simulink subsystem "sensorModels"  (R2026a)
settings: Solver=VariableStepAuto
values from neighbouring files (symbols this model uses):
  envParams : value not decoded    [plantParams.sldd]
  sensorParams : value not decoded    [plantParams.sldd]
undefined symbols (not defined in the file or in its folder): WMM2025
libraries: simulink x7, matrix_library x3, aerolibgravity2 x1
settings Model: DataDictionary=plantParams.sldd  EnableAccessToBaseWorkspace=off  Creator=nathanscott  LastModifiedBy=nathanscott

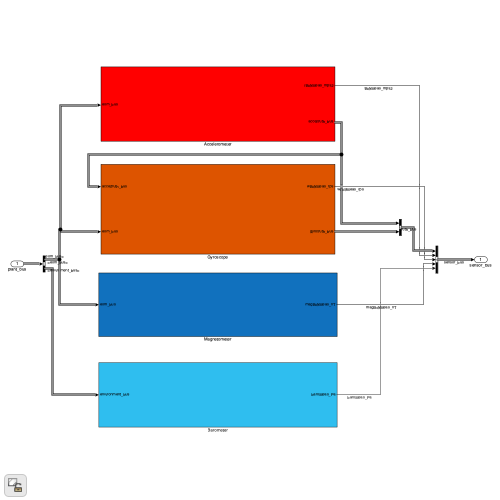
[thumbnail: Simulink's stored preview of the top-level diagram]
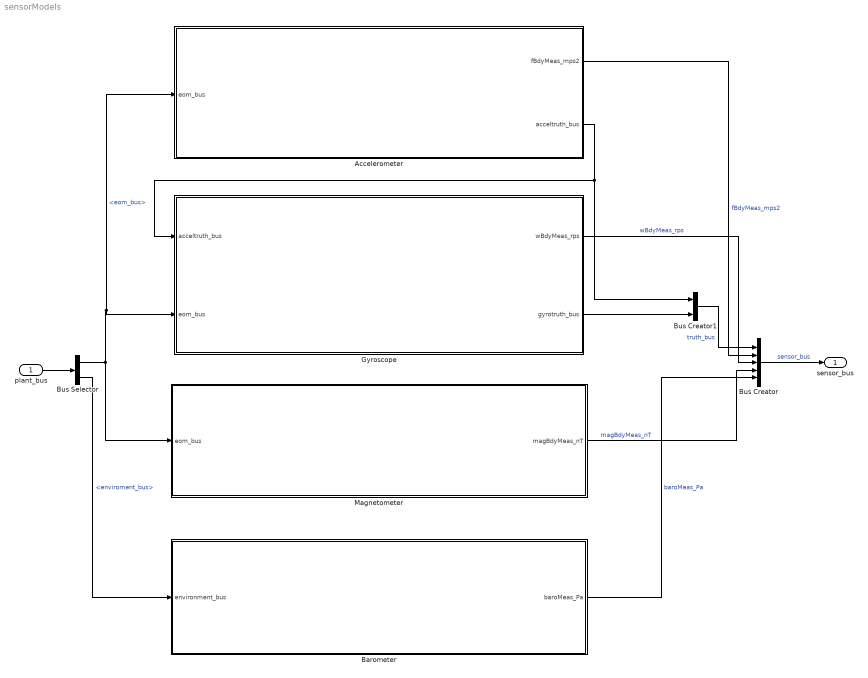
== system sensorModels ==
  plant_bus : Inport
  Accelerometer : Subsystem
  Barometer : Subsystem
  Bus Creator : BusCreator  Inputs=5
  Bus Creator1 : BusCreator  Inputs=2
  Bus Selector : BusSelector  OutputSignals=eom_bus,enviroment_bus
  Gyroscope : Subsystem
  Magnetometer : Subsystem
  sensor_bus : Outport
  wires:
  Bus Creator/1 -> sensor_bus/1  "sensor_bus"
  Accelerometer/1(fBdyMeas_mps2) -> Bus Creator/2  "fBdyMeas_mps2"
  Gyroscope/1(wBdyMeas_rps) -> Bus Creator/3  "wBdyMeas_rps"
  Magnetometer/1(magBdyMeas_nT) -> Bus Creator/4  "magBdyMeas_nT"
  Barometer/1(baroMeas_Pa) -> Bus Creator/5  "baroMeas_Pa"
  plant_bus/1 -> Bus Selector/1
  Bus Selector/2 -> Barometer/1(environment_bus)  "<enviroment_bus>"
  Bus Selector/1 -> Gyroscope/2(eom_bus), Accelerometer/1(eom_bus), Magnetometer/1(eom_bus)  "<eom_bus>"
  Accelerometer/2(acceltruth_bus) -> Gyroscope/1(acceltruth_bus), Bus Creator1/1
  Gyroscope/2(gyrotruth_bus) -> Bus Creator1/2
  Bus Creator1/1 -> Bus Creator/1  "truth_bus"

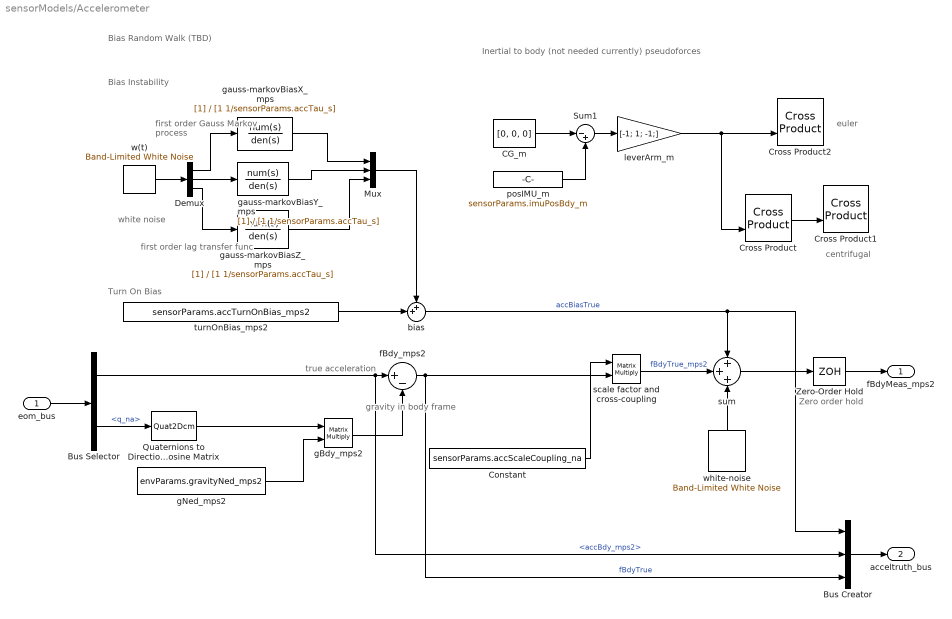
== system sensorModels/Accelerometer ==
  note: Bias Random Walk (TBD)
  note: gravity in body frame
  note: Bias Instability
  note: Turn On Bias
  note: white noise
  note: first order Gauss Markov process
  note: first order lag transfer func
  note: true acceleration
  note: centrifugal
  note: euler
  note: Inertial to body (not needed currently) pseudoforces
  note: Zero order hold
  eom_bus : Inport
  Bus Creator : BusCreator  Inputs=3
  Bus Selector : BusSelector  OutputSignals=accBdy_mps2,q_na
  CG_m : Constant  Value=[0, 0, 0]
  Constant : Constant  Value=sensorParams.accScaleCoupling_na
  Cross Product : matrix_library/Cross Product
  Cross Product1 : matrix_library/Cross Product
  Cross Product2 : matrix_library/Cross Product
  Demux : Demux  Outputs=3
  Mux : Mux  Inputs=3
  Quaternions to Direction Cosine Matrix : Quat2Dcm
  Sum1 : Sum  Inputs=|-+
  Zero-Order Hold : ZeroOrderHold  SampleTime=-1
  bias : Sum  Inputs=++|
  fBdy_mps2 : Sum  Inputs=|+-
  gBdy_mps2 : Product  Multiplication=Matrix(*)
  gNed_mps2 : Constant  Value=envParams.gravityNed_mps2
  gauss-markovBiasX_mps : TransferFcn  Denominator=[1 1/sensorParams.accTau_s]
  gauss-markovBiasY_mps : TransferFcn  Denominator=[1 1/sensorParams.accTau_s]
  gauss-markovBiasZ_mps : TransferFcn  Denominator=[1 1/sensorParams.accTau_s]
  leverArm_m : Gain  Gain=[-1; 1; -1;]
  posIMU_m : Constant  Value=sensorParams.imuPosBdy_m
  scale factor and cross-coupling : Product  Multiplication=Matrix(*)
  sum : Sum  Inputs=+++
  turnOnBias_mps2 : Constant  Value=sensorParams.accTurnOnBias_mps2
  w(t) : simulink/Sources/Band-Limited White Noise  Cov=sensorParams.accPSDGM  Ts=sensorParams.accSampleTime_s  seed=[23341]
  white-noise : simulink/Sources/Band-Limited White Noise  Cov=sensorParams.accPSDWhite  Ts=sensorParams.accSampleTime_s  seed=[23341]
  fBdyMeas_mps2 : Outport
  acceltruth_bus : Outport  Port=2
  wires:
  Bus Creator/1 -> acceltruth_bus/1
  white-noise/1 -> sum/3
  scale factor and cross-coupling/1 -> sum/2  "fBdyTrue_mps2"
  bias/1 -> Bus Creator/1, sum/1  "accBiasTrue"
  fBdy_mps2/1 -> Bus Creator/3, scale factor and cross-coupling/2  "fBdyTrue"
  gBdy_mps2/1 -> fBdy_mps2/2
  Bus Selector/1 -> fBdy_mps2/1, Bus Creator/2  "<accBdy_mps2>"
  turnOnBias_mps2/1 -> bias/2
  Mux/1 -> bias/1
  Zero-Order Hold/1 -> fBdyMeas_mps2/1
  sum/1 -> Zero-Order Hold/1
  Demux/3 -> gauss-markovBiasZ_mps/1
  Demux/2 -> gauss-markovBiasY_mps/1
  Demux/1 -> gauss-markovBiasX_mps/1
  gauss-markovBiasX_mps/1 -> Mux/1
  gauss-markovBiasY_mps/1 -> Mux/2
  gauss-markovBiasZ_mps/1 -> Mux/3
  w(t)/1 -> Demux/1
  posIMU_m/1 -> Sum1/2
  gNed_mps2/1 -> gBdy_mps2/2
  Sum1/1 -> leverArm_m/1
  Quaternions to Direction Cosine Matrix/1 -> gBdy_mps2/1
  Cross Product/1 -> Cross Product1/2
  Bus Selector/2 -> Quaternions to Direction Cosine Matrix/1  "<q_na>"
  eom_bus/1 -> Bus Selector/1
  CG_m/1 -> Sum1/1
  leverArm_m/1 -> Cross Product2/2, Cross Product/2
  Constant/1 -> scale factor and cross-coupling/1

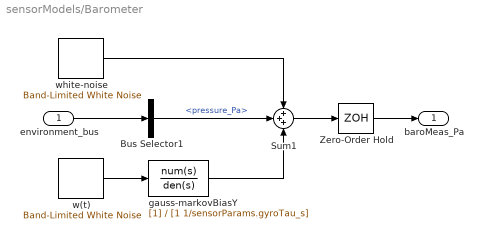
== system sensorModels/Barometer ==
  environment_bus : Inport
  Bus Selector1 : BusSelector  OutputSignals=pressure_Pa
  Sum1 : Sum  Inputs=+++
  Zero-Order Hold : ZeroOrderHold  SampleTime=-1
  gauss-markovBiasY : TransferFcn  Denominator=[1 1/sensorParams.gyroTau_s]
  w(t) : simulink/Sources/Band-Limited White Noise  Cov=sensorParams.baroPSDGM  Ts=sensorParams.baroSampleTime_s  seed=[23341]
  white-noise : simulink/Sources/Band-Limited White Noise  Cov=sensorParams.baroPSDWhite  Ts=sensorParams.baroSampleTime_s  seed=[23341]
  baroMeas_Pa : Outport
  wires:
  w(t)/1 -> gauss-markovBiasY/1
  Sum1/1 -> Zero-Order Hold/1
  gauss-markovBiasY/1 -> Sum1/3
  white-noise/1 -> Sum1/1
  Zero-Order Hold/1 -> baroMeas_Pa/1
  Bus Selector1/1 -> Sum1/2  "<pressure_Pa>"
  environment_bus/1 -> Bus Selector1/1

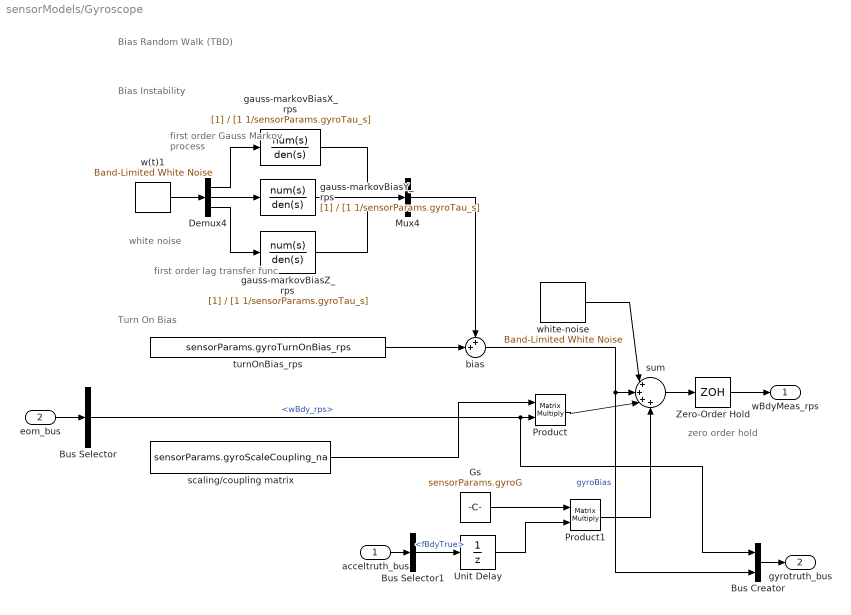
== system sensorModels/Gyroscope ==
  note: first order Gauss Markov process
  note: first order lag transfer func
  note: Bias Random Walk (TBD)
  note: Bias Instability
  note: white noise
  note: Turn On Bias
  note: zero order hold
  acceltruth_bus : Inport
  eom_bus : Inport  Port=2
  Bus Creator : BusCreator  Inputs=2
  Bus Selector : BusSelector  OutputSignals=wBdy_rps
  Bus Selector1 : BusSelector  OutputSignals=fBdyTrue
  Demux4 : Demux  Outputs=3
  Gs : Constant  Value=sensorParams.gyroG
  Mux4 : Mux  Inputs=3
  Product : Product  Multiplication=Matrix(*)
  Product1 : Product  Multiplication=Matrix(*)
  Unit Delay : UnitDelay  SampleTime=-1
  Zero-Order Hold : ZeroOrderHold  SampleTime=-1
  bias : Sum  Inputs=++|
  gauss-markovBiasX_rps : TransferFcn  Denominator=[1 1/sensorParams.gyroTau_s]
  gauss-markovBiasY_rps : TransferFcn  Denominator=[1 1/sensorParams.gyroTau_s]
  gauss-markovBiasZ_rps : TransferFcn  Denominator=[1 1/sensorParams.gyroTau_s]
  scaling/coupling matrix : Constant  Value=sensorParams.gyroScaleCoupling_na
  sum : Sum  Inputs=|++++
  turnOnBias_rps : Constant  Value=sensorParams.gyroTurnOnBias_rps
  w(t)1 : simulink/Sources/Band-Limited White Noise  Cov=sensorParams.gyroPSDGM  Ts=sensorParams.gyroSampleTime_s  seed=[23341]
  white-noise : simulink/Sources/Band-Limited White Noise  Cov=sensorParams.gyroPSDWhite  Ts=sensorParams.gyroSampleTime_s  seed=[23341]
  wBdyMeas_rps : Outport
  gyrotruth_bus : Outport  Port=2
  wires:
  Bus Creator/1 -> gyrotruth_bus/1
  Bus Selector1/1 -> Unit Delay/1  "<fBdyTrue>"
  acceltruth_bus/1 -> Bus Selector1/1
  Product1/1 -> sum/4
  Unit Delay/1 -> Product1/2
  Product/1 -> sum/3
  white-noise/1 -> sum/1
  Mux4/1 -> bias/1
  gauss-markovBiasY_rps/1 -> Mux4/2
  Demux4/1 -> gauss-markovBiasX_rps/1
  turnOnBias_rps/1 -> bias/2
  Demux4/2 -> gauss-markovBiasY_rps/1
  gauss-markovBiasX_rps/1 -> Mux4/1
  Demux4/3 -> gauss-markovBiasZ_rps/1
  w(t)1/1 -> Demux4/1
  gauss-markovBiasZ_rps/1 -> Mux4/3
  Gs/1 -> Product1/1
  scaling/coupling matrix/1 -> Product/1
  Bus Selector/1 -> Product/2, Bus Creator/1  "<wBdy_rps>"
  eom_bus/1 -> Bus Selector/1
  sum/1 -> Zero-Order Hold/1
  Zero-Order Hold/1 -> wBdyMeas_rps/1
  bias/1 -> Bus Creator/2, sum/2  "gyroBias"

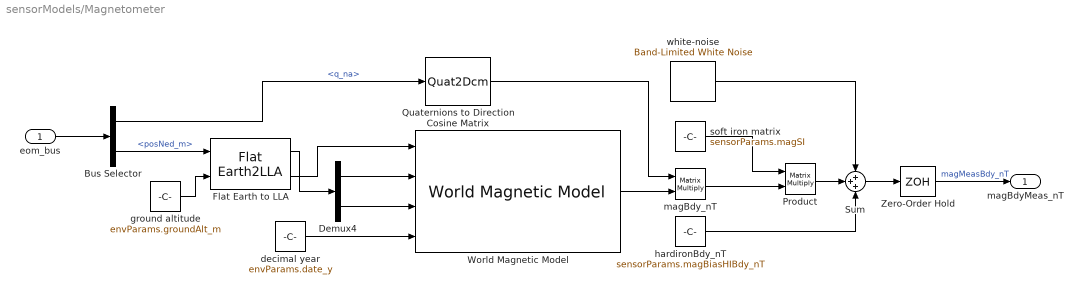
== system sensorModels/Magnetometer ==
  eom_bus : Inport
  Bus Selector : BusSelector  OutputSignals=q_na,posNed_m
  Demux4 : Demux  Outputs=2
  Flat Earth to LLA : FlatEarth2LLA
  Product : Product  Multiplication=Matrix(*)
  Quaternions to Direction Cosine Matrix : Quat2Dcm
  Sum : Sum  Inputs=+++
  World Magnetic Model : aerolibgravity2/World Magnetic Model  model=WMM2025 (2025-2030)  customFile='WMM2025.COF'  units=Metric (MKS)  time_in=on  month=January  day=1  year=2025  action=Error  h_out=off  dec_out=off  inc_out=off  ti_out=off
  Zero-Order Hold : ZeroOrderHold  SampleTime=-1
  decimal year : Constant  Value=envParams.date_y
  ground altitude : Constant  Value=envParams.groundAlt_m
  hardironBdy_nT : Constant  Value=sensorParams.magBiasHIBdy_nT
  magBdy_nT : Product  Multiplication=Matrix(*)
  soft iron matrix : Constant  Value=sensorParams.magSI
  white-noise : simulink/Sources/Band-Limited White Noise  Cov=sensorParams.magPSDWhite  Ts=sensorParams.magSampleTime_s  seed=[23341]
  magBdyMeas_nT : Outport
  wires:
  Zero-Order Hold/1 -> magBdyMeas_nT/1  "magMeasBdy_nT"
  Sum/1 -> Zero-Order Hold/1
  Product/1 -> Sum/2
  white-noise/1 -> Sum/1
  hardironBdy_nT/1 -> Sum/3
  magBdy_nT/1 -> Product/2
  soft iron matrix/1 -> Product/1
  World Magnetic Model/1 -> magBdy_nT/2
  Quaternions to Direction Cosine Matrix/1 -> magBdy_nT/1
  Bus Selector/1 -> Quaternions to Direction Cosine Matrix/1  "<q_na>"
  decimal year/1 -> World Magnetic Model/4
  Flat Earth to LLA/2 -> World Magnetic Model/1
  Demux4/2 -> World Magnetic Model/3
  Demux4/1 -> World Magnetic Model/2
  Flat Earth to LLA/1 -> Demux4/1
  ground altitude/1 -> Flat Earth to LLA/2
  Bus Selector/2 -> Flat Earth to LLA/1  "<posNed_m>"
  eom_bus/1 -> Bus Selector/1
